simulink model "l3"  (R2012b)
settings: Solver=ode45  StartTime=0.0  StopTime=480  RelTol=1e-3
undefined symbols (not defined in the file): des, gcbh
settings Model: Creator=gick  LastModifiedBy=gick

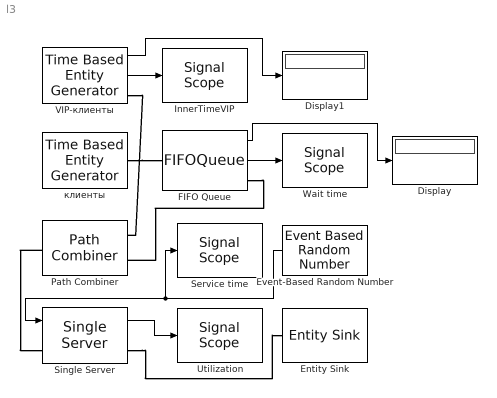
== system l3 ==
  Display : Display
  Display1 : Display
  Entity Sink : EntitySink
  Event-Based Random Number : EventBasedRandomNumber  Distribution=Uniform  meanExp=15  minUnif=5  maxUnif=16  Seed=1234
  FIFO Queue : FIFOQueue  Capacity=20  StatNumberDeparted=on  StatAverageWait=on
      settings: OutputPortMap=o0,o2
  InnerTimeVIP : SignalScope  LoadFcn=des.scope.CallbackSupport('seLoadFcn',gcbh)  StartFcn=des.scope.CallbackSupport('seStartFcn',gcbh)  StopFcn=des.scope.CallbackSupport('seStopFcn',gcbh)  ShowCountPlotted=on
      settings: CopyFcn=des.scope.CallbackSupport('seCopyFcn',gcbh)  DeleteFcn=des.scope.CallbackSupport('seDeleteFcn',gcbh)  PreSaveFcn=des.scope.CallbackSupport('sePreSaveFcn',gcbh)  NameChangeFcn=des.scope.CallbackSupport('seNameChangeFcn',gcbh)  OpenFcn=des.scope.CallbackSupport('seOpenFcn',gcbh)
  Path Combiner : PathCombiner  NumberInputPorts=2
  Service time : SignalScope  LoadFcn=des.scope.CallbackSupport('seLoadFcn',gcbh)  StartFcn=des.scope.CallbackSupport('seStartFcn',gcbh)  StopFcn=des.scope.CallbackSupport('seStopFcn',gcbh)  ShowCountPlotted=on
      settings: CopyFcn=des.scope.CallbackSupport('seCopyFcn',gcbh)  DeleteFcn=des.scope.CallbackSupport('seDeleteFcn',gcbh)  PreSaveFcn=des.scope.CallbackSupport('sePreSaveFcn',gcbh)  NameChangeFcn=des.scope.CallbackSupport('seNameChangeFcn',gcbh)  OpenFcn=des.scope.CallbackSupport('seOpenFcn',gcbh)
  Single Server : SingleServer  ServiceTimeFrom=Signal port t  AttributeName=servtime  StatUtilization=on
      settings: OutputPortMap=o5
  Utilization : SignalScope  LoadFcn=des.scope.CallbackSupport('seLoadFcn',gcbh)  StartFcn=des.scope.CallbackSupport('seStartFcn',gcbh)  StopFcn=des.scope.CallbackSupport('seStopFcn',gcbh)  ShowCountPlotted=on
      settings: CopyFcn=des.scope.CallbackSupport('seCopyFcn',gcbh)  DeleteFcn=des.scope.CallbackSupport('seDeleteFcn',gcbh)  PreSaveFcn=des.scope.CallbackSupport('sePreSaveFcn',gcbh)  NameChangeFcn=des.scope.CallbackSupport('seNameChangeFcn',gcbh)  OpenFcn=des.scope.CallbackSupport('seOpenFcn',gcbh)
  VIP-клиенты : TimeBasedEntityGenerator  Distribution=Exponential  Mean=60  StatNumberDeparted=on  StatAverageIntergenerationTime=on
      settings: OutputPortMap=o0,o2
  Wait time : SignalScope  LoadFcn=des.scope.CallbackSupport('seLoadFcn',gcbh)  StartFcn=des.scope.CallbackSupport('seStartFcn',gcbh)  StopFcn=des.scope.CallbackSupport('seStopFcn',gcbh)  ShowCountPlotted=on
      settings: CopyFcn=des.scope.CallbackSupport('seCopyFcn',gcbh)  DeleteFcn=des.scope.CallbackSupport('seDeleteFcn',gcbh)  PreSaveFcn=des.scope.CallbackSupport('sePreSaveFcn',gcbh)  NameChangeFcn=des.scope.CallbackSupport('seNameChangeFcn',gcbh)  OpenFcn=des.scope.CallbackSupport('seOpenFcn',gcbh)
  клиенты : TimeBasedEntityGenerator  Distribution=Exponential  Mean=15
  wires:
  FIFO Queue/2 -> Wait time/1
  Single Server/1 -> Utilization/1
  Event-Based Random Number/1 -> Service time/1, Single Server/1
  VIP-клиенты/1 -> Display1/1
  VIP-клиенты/2 -> InnerTimeVIP/1
  FIFO Queue/1 -> Display/1
  connections:
  Single Server/RConn1 -- Entity Sink/LConn1
  VIP-клиенты/RConn1 -- Path Combiner/LConn1
  клиенты/RConn1 -- FIFO Queue/LConn1
  Path Combiner/RConn1 -- Single Server/LConn1
  FIFO Queue/RConn1 -- Path Combiner/LConn2
